simulink model "timer_8bit"  (R2016a)
settings: Solver=VariableStepAuto  StartTime=0.0  StopTime=514  RelTol=1e-3
libraries: simulink_extras x9
settings Model: Creator=Cosmin  LastModifiedBy=Cosmin

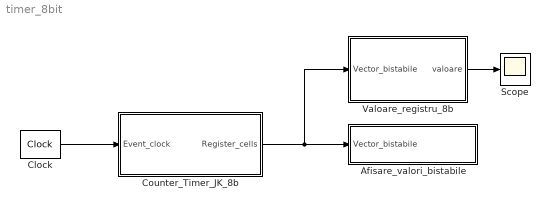
== system timer_8bit ==
  Afisare_valori_bistabile : Subsystem
  Clock : simulink_extras/Flip Flops/Clock  period=2
  Counter_Timer_JK_8b : Subsystem
  Scope : Scope
  Valoare_registru_8b : Subsystem
  wires:
  Valoare_registru_8b/1(valoare) -> Scope/1
  Counter_Timer_JK_8b/1(Register_cells) -> Afisare_valori_bistabile/1(Vector_bistabile), Valoare_registru_8b/1(Vector_bistabile)
  Clock/1 -> Counter_Timer_JK_8b/1(Event_clock)

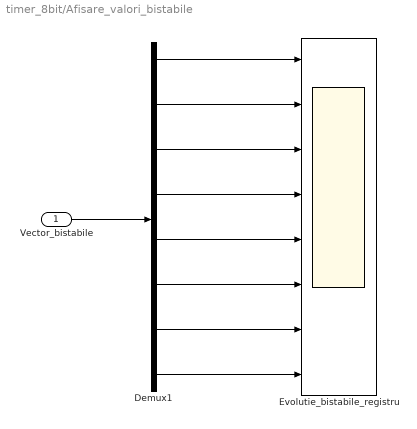
== system timer_8bit/Afisare_valori_bistabile ==
  Vector_bistabile : Inport
  Demux1 : Demux  Outputs=8
  Evolutie_bistabile_registru : Scope  NumInputPorts=8
  wires:
  Vector_bistabile/1 -> Demux1/1
  Demux1/4 -> Evolutie_bistabile_registru/4
  Demux1/2 -> Evolutie_bistabile_registru/2
  Demux1/1 -> Evolutie_bistabile_registru/1
  Demux1/3 -> Evolutie_bistabile_registru/3
  Demux1/7 -> Evolutie_bistabile_registru/7
  Demux1/5 -> Evolutie_bistabile_registru/5
  Demux1/6 -> Evolutie_bistabile_registru/6
  Demux1/8 -> Evolutie_bistabile_registru/8

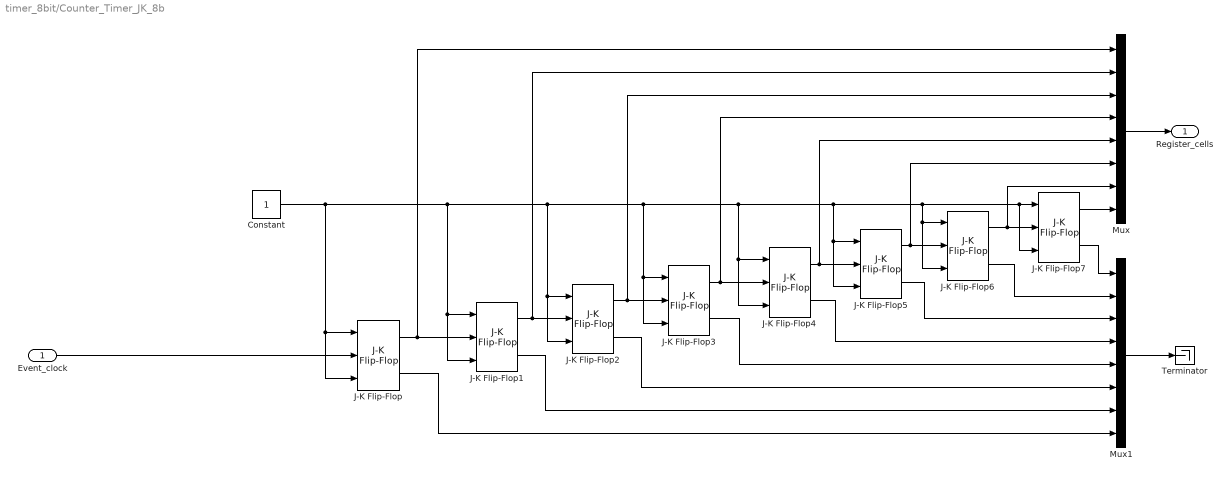
== system timer_8bit/Counter_Timer_JK_8b ==
  Event_clock : Inport
  Constant : Constant  OutDataTypeStr=boolean
  J-K Flip-Flop{,1..7} (8 alike) : simulink_extras/Flip Flops/J-K Flip-Flop  initial_condition=0
  Mux : Mux  Inputs=8
  Mux1 : Mux  Inputs=8
  Terminator : Terminator
  Register_cells : Outport
  wires:
  J-K Flip-Flop6/1 -> Mux/7, J-K Flip-Flop7/2
  J-K Flip-Flop7/1 -> Mux/8
  J-K Flip-Flop/1 -> Mux/1, J-K Flip-Flop1/2
  Constant/1 -> J-K Flip-Flop/3, J-K Flip-Flop/1, J-K Flip-Flop1/3, J-K Flip-Flop1/1, J-K Flip-Flop2/3, J-K Flip-Flop2/1, J-K Flip-Flop3/3, J-K Flip-Flop3/1, J-K Flip-Flop4/3, J-K Flip-Flop4/1, J-K Flip-Flop7/3, J-K Flip-Flop7/1, J-K Flip-Flop6/3, J-K Flip-Flop6/1, J-K Flip-Flop5/3, J-K Flip-Flop5/1
  J-K Flip-Flop5/1 -> Mux/6, J-K Flip-Flop6/2
  J-K Flip-Flop2/1 -> Mux/3, J-K Flip-Flop3/2
  J-K Flip-Flop1/1 -> Mux/2, J-K Flip-Flop2/2
  J-K Flip-Flop7/2 -> Mux1/1
  J-K Flip-Flop4/1 -> Mux/5, J-K Flip-Flop5/2
  Event_clock/1 -> J-K Flip-Flop/2
  Mux/1 -> Register_cells/1
  J-K Flip-Flop3/1 -> Mux/4, J-K Flip-Flop4/2
  J-K Flip-Flop6/2 -> Mux1/2
  J-K Flip-Flop5/2 -> Mux1/3
  J-K Flip-Flop4/2 -> Mux1/4
  J-K Flip-Flop3/2 -> Mux1/5
  J-K Flip-Flop2/2 -> Mux1/6
  J-K Flip-Flop1/2 -> Mux1/7
  J-K Flip-Flop/2 -> Mux1/8
  Mux1/1 -> Terminator/1

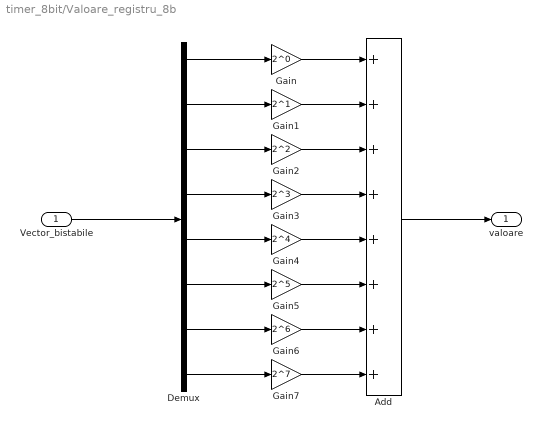
== system timer_8bit/Valoare_registru_8b ==
  Vector_bistabile : Inport
  Add : Sum  Inputs=++++++++
  Demux : Demux  Outputs=8
  Gain : Gain  Gain=2^0  OutDataTypeStr=uint8
  Gain1 : Gain  Gain=2^1  OutDataTypeStr=uint8
  Gain2 : Gain  Gain=2^2  OutDataTypeStr=uint8
  Gain3 : Gain  Gain=2^3  OutDataTypeStr=uint8
  Gain4 : Gain  Gain=2^4  OutDataTypeStr=uint8
  Gain5 : Gain  Gain=2^5  OutDataTypeStr=uint8
  Gain6 : Gain  Gain=2^6  OutDataTypeStr=uint8
  Gain7 : Gain  Gain=2^7  OutDataTypeStr=uint8
  valoare : Outport
  wires:
  Demux/1 -> Gain/1
  Demux/6 -> Gain5/1
  Demux/7 -> Gain6/1
  Demux/2 -> Gain1/1
  Demux/5 -> Gain4/1
  Gain5/1 -> Add/6
  Gain6/1 -> Add/7
  Gain2/1 -> Add/3
  Gain4/1 -> Add/5
  Gain3/1 -> Add/4
  Gain7/1 -> Add/8
  Gain1/1 -> Add/2
  Gain/1 -> Add/1
  Vector_bistabile/1 -> Demux/1
  Demux/3 -> Gain2/1
  Demux/4 -> Gain3/1
  Demux/8 -> Gain7/1
  Add/1 -> valoare/1
